simulink model "modelSuperLUCAb"  (R2015b)
settings: Solver=ode45  SolverMode=SingleTasking  StartTime=0.0  StopTime=10.0  RelTol=1e-3
values from neighbouring files (symbols this model uses):
  T21 = [cos(theta2) -sin(theta2) 0;sin(theta2) cos(theta2) 0;0 0 1]    [pourDaniel.m]    (also in twodofarm.m)
undefined symbols (not defined in the file or in its folder): Jh1, Jh2, Jp, mh2, mp
libraries: cstblocks x2
settings Model: Creator=d.alazard  LastModifiedBy=d.alazard
settings DataIOCC: SaveFormat=Array
settings OptimizationCC: BlockReduction=off  BooleanDataType=off
settings DebuggingCC: SaveWithParameterizedLinksMsg=none  UnderspecifiedInitializationDetection=Classic  MergeDetectMultiDrivingBlocksExec=none  SignalResolutionControl=TryResolveAllWithWarning
settings HardwareCC: ProdBitPerPointer=32  ProdLargestAtomicFloat=None  ProdIntDivRoundTo=Undefined  ProdEndianess=Unspecified  ProdWordSize=32  ProdHWDeviceType=32-bit Generic  TargetUnknown=on
settings GRTTargetCC: GeneratePreprocessorConditionals=Disable all
settings ConfigComp: CovModelRefEnable=Off  CovSFcnEnable=off

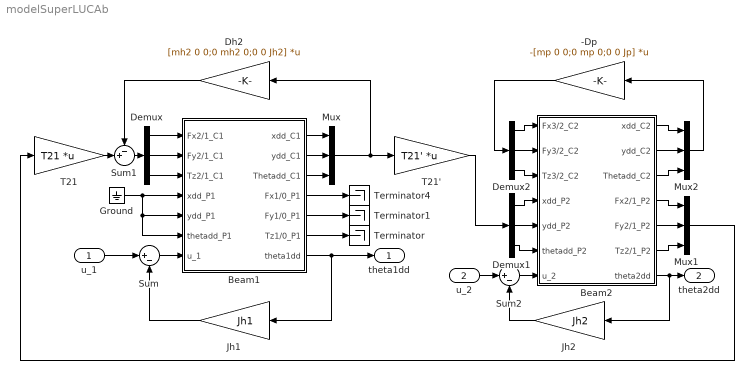
== system modelSuperLUCAb ==
  u_1 : Inport
  u_2 : Inport  Port=2
  -Dp : Gain  Gain=-[mp 0 0;0 mp 0;0 0 Jp]  Multiplication=Matrix(K*u) (u vector)
  Beam1 : Subsystem
  Beam2 : Subsystem
  Demux : Demux  Outputs=3
  Demux1 : Demux  Outputs=3
  Demux2 : Demux  Outputs=3
  Dh2 : Gain  Gain=[mh2 0 0;0 mh2 0;0 0 Jh2]  Multiplication=Matrix(K*u) (u vector)
  Ground : Ground
  Jh1 : Gain  Gain=Jh1
  Jh2 : Gain  Gain=Jh2
  Mux : Mux  Inputs=3
  Mux1 : Mux  Inputs=3
  Mux2 : Mux  Inputs=3
  Sum : Sum  Inputs=|+-
  Sum1 : Sum  Inputs=-+|
  Sum2 : Sum  Inputs=|+-
  T21 : Gain  Gain=T21  Multiplication=Matrix(K*u) (u vector)
  T21' : Gain  Gain=T21'  Multiplication=Matrix(K*u) (u vector)
  Terminator : Terminator
  Terminator1 : Terminator
  Terminator4 : Terminator
  theta1dd : Outport
  theta2dd : Outport  Port=2
  wires:
  Ground/1 -> Beam1/6(thetadd_P1), Beam1/5(ydd_P1), Beam1/4(xdd_P1)
  Beam1/4(Fx1/0_P1) -> Terminator4/1
  Beam1/5(Fy1/0_P1) -> Terminator1/1
  Beam1/6(Tz1/0_P1) -> Terminator/1
  Beam1/7(theta1dd) -> Jh1/1, theta1dd/1
  Beam1/1(xdd_C1) -> Mux/1
  Beam1/2(ydd_C1) -> Mux/2
  Beam2/4(Fx2/1_P2) -> Mux1/1
  Beam2/5(Fy2/1_P2) -> Mux1/2
  Demux/1 -> Beam1/1(Fx2/1_C1)
  Demux/2 -> Beam1/2(Fy2/1_C1)
  Demux1/1 -> Beam2/4(xdd_P2)
  Demux1/2 -> Beam2/5(ydd_P2)
  Beam2/1(xdd_C2) -> Mux2/1
  Beam2/2(ydd_C2) -> Mux2/2
  Beam2/3(Thetadd_C2) -> Mux2/3
  Mux/1 -> Dh2/1, T21'/1
  Beam2/7(theta2dd) -> theta2dd/1, Jh2/1
  Beam1/3(Thetadd_C1) -> Mux/3
  Demux/3 -> Beam1/3(Tz2/1_C1)
  Beam2/6(Tz2/1_P2) -> Mux1/3
  Demux1/3 -> Beam2/6(thetadd_P2)
  T21'/1 -> Demux1/1
  Mux1/1 -> T21/1
  u_1/1 -> Sum/1
  Sum/1 -> Beam1/7(u_1)
  Jh1/1 -> Sum/2
  Sum1/1 -> Demux/1
  T21/1 -> Sum1/2
  Dh2/1 -> Sum1/1
  Mux2/1 -> -Dp/1
  Demux2/1 -> Beam2/1(Fx3/2_C2)
  Demux2/2 -> Beam2/2(Fy3/2_C2)
  Demux2/3 -> Beam2/3(Tz3/2_C2)
  -Dp/1 -> Demux2/1
  Sum2/1 -> Beam2/7(u_2)
  u_2/1 -> Sum2/1
  Jh2/1 -> Sum2/2

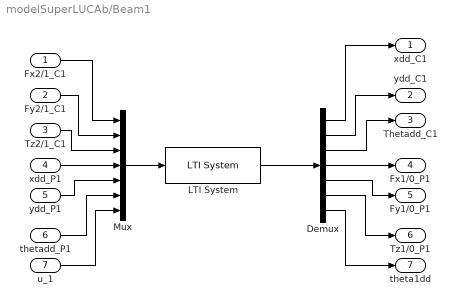
== system modelSuperLUCAb/Beam1 ==
  Fx2/1_C1 : Inport
  Fy2/1_C1 : Inport  Port=2
  Tz2/1_C1 : Inport  Port=3
  xdd_P1 : Inport  Port=4
  ydd_P1 : Inport  Port=5
  thetadd_P1 : Inport  Port=6
  u_1 : Inport  Port=7
  Demux : Demux  Outputs=7
  LTI System : cstblocks/LTI System  sys=Mbm1_7  IC=[]
  Mux : Mux  Inputs=7
  xdd_C1 : Outport
  ydd_C1 : Outport  Port=2
  Thetadd_C1 : Outport  Port=3
  Fx1/0_P1 : Outport  Port=4
  Fy1/0_P1 : Outport  Port=5
  Tz1/0_P1 : Outport  Port=6
  theta1dd : Outport  Port=7
  wires:
  LTI System/1 -> Demux/1
  Mux/1 -> LTI System/1
  Fx2/1_C1/1 -> Mux/1
  Fy2/1_C1/1 -> Mux/2
  Tz2/1_C1/1 -> Mux/3
  xdd_P1/1 -> Mux/4
  ydd_P1/1 -> Mux/5
  thetadd_P1/1 -> Mux/6
  u_1/1 -> Mux/7
  Demux/1 -> xdd_C1/1
  Demux/2 -> ydd_C1/1
  Demux/3 -> Thetadd_C1/1
  Demux/4 -> Fx1/0_P1/1
  Demux/5 -> Fy1/0_P1/1
  Demux/6 -> Tz1/0_P1/1
  Demux/7 -> theta1dd/1

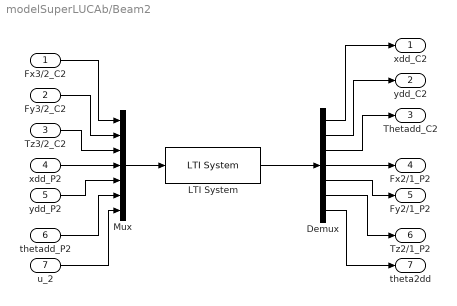
== system modelSuperLUCAb/Beam2 ==
  Fx3/2_C2 : Inport
  Fy3/2_C2 : Inport  Port=2
  Tz3/2_C2 : Inport  Port=3
  xdd_P2 : Inport  Port=4
  ydd_P2 : Inport  Port=5
  thetadd_P2 : Inport  Port=6
  u_2 : Inport  Port=7
  Demux : Demux  Outputs=7
  LTI System : cstblocks/LTI System  sys=Mbm1_7  IC=[]
  Mux : Mux  Inputs=7
  xdd_C2 : Outport
  ydd_C2 : Outport  Port=2
  Thetadd_C2 : Outport  Port=3
  Fx2/1_P2 : Outport  Port=4
  Fy2/1_P2 : Outport  Port=5
  Tz2/1_P2 : Outport  Port=6
  theta2dd : Outport  Port=7
  wires:
  Mux/1 -> LTI System/1
  LTI System/1 -> Demux/1
  Demux/1 -> xdd_C2/1
  Demux/2 -> ydd_C2/1
  Demux/3 -> Thetadd_C2/1
  Demux/4 -> Fx2/1_P2/1
  Demux/5 -> Fy2/1_P2/1
  Demux/6 -> Tz2/1_P2/1
  Demux/7 -> theta2dd/1
  xdd_P2/1 -> Mux/4
  Tz3/2_C2/1 -> Mux/3
  Fy3/2_C2/1 -> Mux/2
  Fx3/2_C2/1 -> Mux/1
  ydd_P2/1 -> Mux/5
  thetadd_P2/1 -> Mux/6
  u_2/1 -> Mux/7
